simulink library "nmm"  (R2021b)
settings: Solver=VariableStepAuto  StartTime=0.0  StopTime=10.0  RelTol=1e-3
undefined symbols (not defined in the file or in its folder): ENUM_NMMCURRENTSTATE_SLEEP, ENUM_SYSNMMSTA_NORMAL, ENUM_SYSNMMSTA_READYSLEEP, FALSE, KNMM_NoNMIdDebounce_s, KNMM_NrmStaDelay_s, KNMM_RdySlpStaDelay_s, KPMM_HVBattSOCThd_pct, slcm, TRUE, ZERO_INT
libraries: hcu_lib x2, simulink x1
settings Model: Creator=13615  LastModifiedBy=FVT22063
settings SolverCC: AlgebraicLoopSolver=TrustRegion
settings DataIOCC: SaveFormat=Array  SignalLoggingSaveFormat=ModelDataLogs  ReturnWorkspaceOutputs=off
settings OptimizationCC: BlockReduction=off  BooleanDataType=off
settings DebuggingCC: SaveWithParameterizedLinksMsg=none  UnderspecifiedInitializationDetection=Classic  MergeDetectMultiDrivingBlocksExec=none  SignalResolutionControl=TryResolveAllWithWarning  SFMachineParentedDataDiag=warning  ArithmeticOperatorsInVariantConditions=warning
settings HardwareCC: TargetUnknown=on
settings ModelReferenceCC: PropagateSignalLabelsOutOfModel=off
settings SFSimCC: SimUseLocalCustomCode=off  CustomCodeUndefinedFunction=UseInterfaceOnly
settings RTWCC: RTWUseLocalCustomCode=off
settings ConfigComp: CovMetricSettings=dw  CovSaveCumulativeToWorkspaceVar=on  CovSaveSingleToWorkspaceVar=on

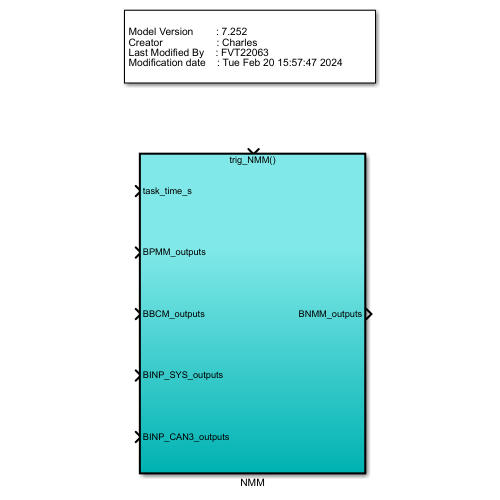
[thumbnail: Simulink's stored preview of the top-level diagram]
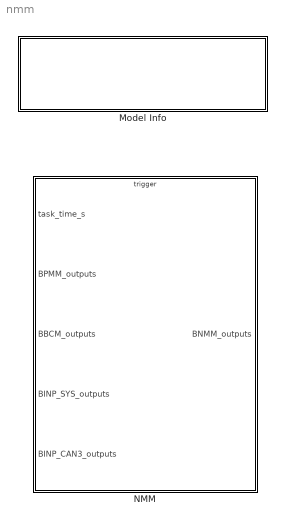
== system nmm ==
  Model Info : Subsystem  LoadFcn=slcm LoadBlock;  InitFcn=slcm('UpdateAllCMBlocksInThisModelInit')  mask(CMBlock){InitialSaveTempField=, InitialBlockCM=None, BlockCM=None, Frame=on, SaveTempField=, DisplayStringWithTags=|, MaskDisplayString=Model Version        : 7.287\nCreator                   : Charles\nLast Modified By    : FVT22063\nModification date    : Tue Aug 27 16:39:44 2024, HorizontalTextAlignment=Left, LeftAlignmentValue=0.02, SourceBlockDiagram=pmm, TagMaxNumber=20, CMTag1=, CMTag2=, CMTag3=, CMTag4=, CMTag5=, CMTag6=, CMTag7=, CMTag8=, CMTag9=, CMTag10=, CMTag11=, CMTag12=, CMTag13=, CMTag14=, CMTag15=, CMTag16=, CMTag17=, CMTag18=, CMTag19=, CMTag20=}
      mask DisplayStringWithTags=|
      | Model Version        : %<ModelVersion>
      | Creator                   : Charles
      | Last Modified By    : %<LastModifiedBy>
      | Modification date    : %<LastModificationDate>
      mask help: This block allows revision control information to be displayed within the model.
      settings: CopyFcn=slcm CopyBlock;  DeleteFcn=slcm Cancel;  PostSaveFcn=slcm('UpdateAllCMBlocksInThisModel')  NameChangeFcn=slcm Rename;  OpenFcn=slcm
      mask Display: text(str2num(LeftAlignmentValue), 0.5, MaskDisplayString, 'HorizontalAlignment', HorizontalTextAlignment)
  NMM : Subsystem  TreatAsAtomicUnit=on
      settings: RTWSystemCode=Nonreusable function  RTWFcnNameOpts=Use subsystem name  RTWFileNameOpts=Use subsystem name

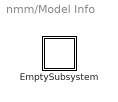
== system nmm/Model Info ==
  EmptySubsystem : Subsystem

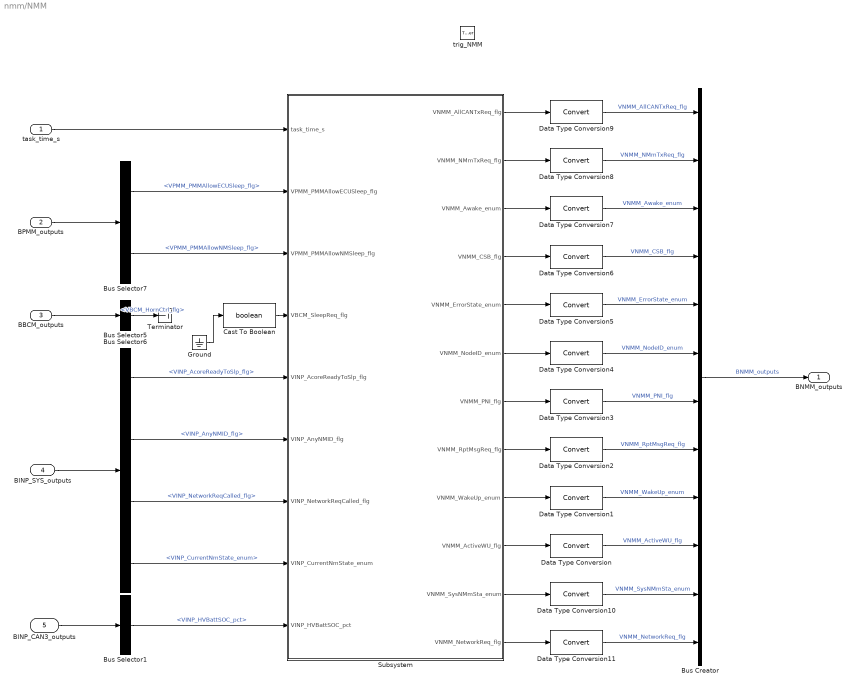
== system nmm/NMM ==
  task_time_s : Inport
  BPMM_outputs : Inport  Port=2  OutDataTypeStr=Bus: BPMM_outputs
  BBCM_outputs : Inport  Port=3  OutDataTypeStr=Bus: BBCM_outputs
  BINP_SYS_outputs : Inport  Port=4  OutDataTypeStr=Bus: BINP_SYS_outputs
  BINP_CAN3_outputs : Inport  Port=5  OutDataTypeStr=Bus: BINP_CAN3_outputs
  trig_NMM : TriggerPort  TriggerType=function-call  VariantControl=(inherit)
  Bus Creator : BusCreator  Inputs=12  OutDataTypeStr=Bus: BNMM_outputs
  Bus Selector1 : BusSelector  OutputSignals=VINP_HVBattSOC_pct
  Bus Selector5 : BusSelector  OutputSignals=VBCM_HornCtrl_flg
  Bus Selector6 : BusSelector  OutputSignals=VINP_AcoreReadyToSlp_flg,VINP_AnyNMID_flg,VINP_NetworkReqCalled_flg,VINP_CurrentNmState_enum
  Bus Selector7 : BusSelector  OutputSignals=VPMM_PMMAllowECUSleep_flg,VPMM_PMMAllowNMSleep_flg
  Cast To Boolean : DataTypeConversion  OutDataTypeStr=boolean
  Data Type Conversion{,1..11} (12 alike) : DataTypeConversion
  Ground : Ground
  Subsystem : Subsystem
  Terminator : Terminator
  BNMM_outputs : Outport  OutDataTypeStr=Bus: BNMM_outputs  LockScale=on
  wires:
  Data Type Conversion9/1 -> Bus Creator/1  "VNMM_AllCANTxReq_flg"
  Data Type Conversion8/1 -> Bus Creator/2  "VNMM_NMmTxReq_flg"
  Data Type Conversion7/1 -> Bus Creator/3  "VNMM_Awake_enum"
  Data Type Conversion6/1 -> Bus Creator/4  "VNMM_CSB_flg"
  Data Type Conversion5/1 -> Bus Creator/5  "VNMM_ErrorState_enum"
  Data Type Conversion4/1 -> Bus Creator/6  "VNMM_NodeID_enum"
  Data Type Conversion3/1 -> Bus Creator/7  "VNMM_PNI_flg"
  Data Type Conversion2/1 -> Bus Creator/8  "VNMM_RptMsgReq_flg"
  Data Type Conversion1/1 -> Bus Creator/9  "VNMM_WakeUp_enum"
  Data Type Conversion/1 -> Bus Creator/10  "VNMM_ActiveWU_flg"
  Bus Creator/1 -> BNMM_outputs/1  "BNMM_outputs"
  Subsystem/10(VNMM_ActiveWU_flg) -> Data Type Conversion/1
  Subsystem/9(VNMM_WakeUp_enum) -> Data Type Conversion1/1
  Subsystem/8(VNMM_RptMsgReq_flg) -> Data Type Conversion2/1
  Subsystem/7(VNMM_PNI_flg) -> Data Type Conversion3/1
  Subsystem/6(VNMM_NodeID_enum) -> Data Type Conversion4/1
  Subsystem/5(VNMM_ErrorState_enum) -> Data Type Conversion5/1
  Subsystem/4(VNMM_CSB_flg) -> Data Type Conversion6/1
  Subsystem/3(VNMM_Awake_enum) -> Data Type Conversion7/1
  Subsystem/2(VNMM_NMmTxReq_flg) -> Data Type Conversion8/1
  Subsystem/1(VNMM_AllCANTxReq_flg) -> Data Type Conversion9/1
  BPMM_outputs/1 -> Bus Selector7/1
  Data Type Conversion10/1 -> Bus Creator/11  "VNMM_SysNMmSta_enum"
  Subsystem/11(VNMM_SysNMmSta_enum) -> Data Type Conversion10/1
  BBCM_outputs/1 -> Bus Selector5/1
  BINP_SYS_outputs/1 -> Bus Selector6/1
  Data Type Conversion11/1 -> Bus Creator/12  "VNMM_NetworkReq_flg"
  Subsystem/12(VNMM_NetworkReq_flg) -> Data Type Conversion11/1
  task_time_s/1 -> Subsystem/1(task_time_s)
  Bus Selector7/2 -> Subsystem/3(VPMM_PMMAllowNMSleep_flg)  "<VPMM_PMMAllowNMSleep_flg>"
  Bus Selector6/2 -> Subsystem/6(VINP_AnyNMID_flg)  "<VINP_AnyNMID_flg>"
  Bus Selector6/1 -> Subsystem/5(VINP_AcoreReadyToSlp_flg)  "<VINP_AcoreReadyToSlp_flg>"
  Bus Selector1/1 -> Subsystem/9(VINP_HVBattSOC_pct)  "<VINP_HVBattSOC_pct>"
  BINP_CAN3_outputs/1 -> Bus Selector1/1
  Bus Selector7/1 -> Subsystem/2(VPMM_PMMAllowECUSleep_flg)  "<VPMM_PMMAllowECUSleep_flg>"
  Bus Selector6/3 -> Subsystem/7(VINP_NetworkReqCalled_flg)  "<VINP_NetworkReqCalled_flg>"
  Bus Selector6/4 -> Subsystem/8(VINP_CurrentNmState_enum)  "<VINP_CurrentNmState_enum>"
  Cast To Boolean/1 -> Subsystem/4(VBCM_SleepReq_flg)
  Ground/1 -> Cast To Boolean/1
  Bus Selector5/1 -> Terminator/1  "<VBCM_HornCtrl_flg>"

== system nmm/Model Info/EmptySubsystem ==

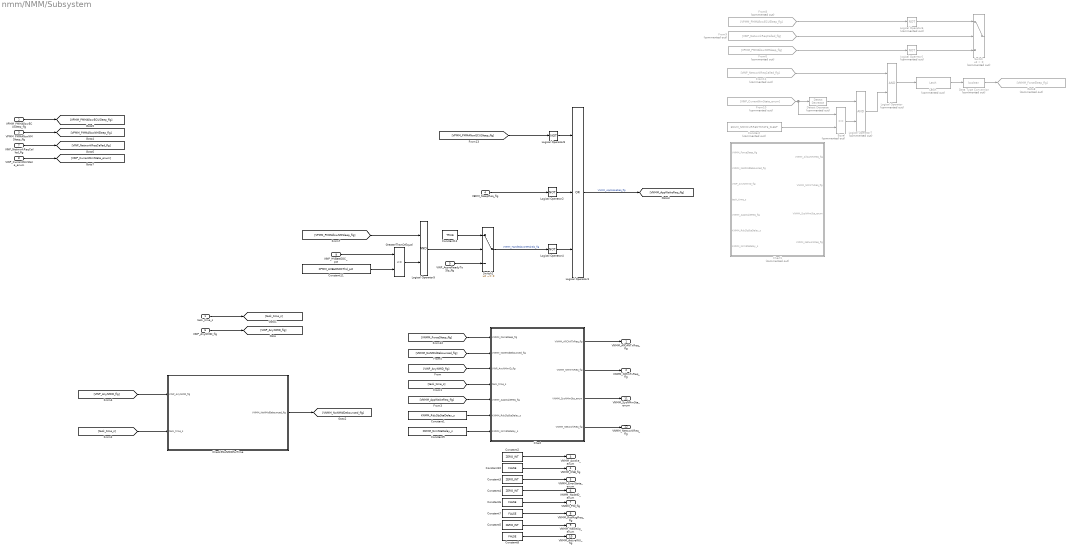
== system nmm/NMM/Subsystem ==
  task_time_s : Inport
  VPMM_PMMAllowECUSleep_flg : Inport  Port=2
  VPMM_PMMAllowNMSleep_flg : Inport  Port=3
  VBCM_SleepReq_flg : Inport  Port=4
  VINP_AcoreReadyToSlp_flg : Inport  Port=5
  VINP_AnyNMID_flg : Inport  Port=6
  VINP_NetworkReqCalled_flg : Inport  Port=7
  VINP_CurrentNmState_enum : Inport  Port=8
  VINP_HVBattSOC_pct : Inport  Port=9
  Chart : Stateflow chart  TreatAsAtomicUnit=on
  Chart1 : Stateflow chart  Commented=on  TreatAsAtomicUnit=on
  CheckIfNoNMIDforTime : Subsystem
  Constant : Constant  Commented=on  Value=ENUM_NMMCURRENTSTATE_SLEEP
  Constant1 : Constant  Value=KNMM_RdySlpStaDelay_s
  Constant{6..8,10} (4 alike) : Constant  Value=FALSE  OutDataTypeStr=boolean
  Constant11 : Constant  Value=KPMM_HVBattSOCThd_pct
  Constant12 : Constant  Value=TRUE
  Constant{2..5} (4 alike) : Constant  Value=ZERO_INT  OutDataTypeStr=uint8
  Constant9 : Constant  Value=KNMM_NrmStaDelay_s
  Data Type Conversion : DataTypeConversion  Commented=on  OutDataTypeStr=boolean
  Detect Decrease : simulink/Logic and Bit Operations/Detect Decrease  Commented=on  vinit=0.0  OutDataTypeStr=boolean
  Equal : RelationalOperator  Commented=on  Operator===  OutDataTypeStr=boolean  RndMeth=Simplest
  From10 : From  Commented=on  GotoTag=VINP_CurrentNmState_enum
  From11 : From  Commented=on  GotoTag=VINP_NetworkReqCalled_flg
  From6 : From  Commented=on  GotoTag=VPMM_PMMAllowNMSleep_flg
  From8 : From  Commented=on  GotoTag=VPMM_PMMAllowECUSleep_flg
  From9 : From  Commented=on  GotoTag=VINP_NetworkReqCalled_flg
  Goto8 : Goto  Commented=on  GotoTag=VNMM_ForceSleep_flg
  GreaterThanOrEqual : RelationalOperator  Operator=<=  OutDataTypeStr=boolean  RndMeth=Simplest
  Latch : hcu_lib/Basic_Blocks/Latch  Commented=on
  Logical Operator : Logic  Commented=on  AllPortsSameDT=off  OutDataTypeStr=boolean
  Logical Operator1 : Logic  Commented=on  Operator=NOT  AllPortsSameDT=off  OutDataTypeStr=boolean
  Logical Operator2 : Logic  Operator=NOT  AllPortsSameDT=off  OutDataTypeStr=boolean
  Logical Operator3 : Logic  Operator=OR  Inputs=3  AllPortsSameDT=off  OutDataTypeStr=boolean
  Logical Operator4 : Logic  Operator=NOT  AllPortsSameDT=off  OutDataTypeStr=boolean
  Logical Operator5 : Logic  AllPortsSameDT=off  OutDataTypeStr=boolean
  Logical Operator6 : Logic  Commented=on  Operator=NOT  AllPortsSameDT=off  OutDataTypeStr=boolean
  Logical Operator7 : Logic  Commented=on  AllPortsSameDT=off  OutDataTypeStr=boolean
  Logical Operator8 : Logic  Operator=NOT  AllPortsSameDT=off  OutDataTypeStr=boolean
  Switch : Switch  Commented=on  Criteria=u2 > Threshold
  Switch2 : Switch  Criteria=u2 ~= 0
  VNMM_AllCANTxReq_flg : Outport
  VNMM_NMmTxReq_flg : Outport  Port=2
  VNMM_Awake_enum : Outport  Port=3
  VNMM_CSB_flg : Outport  Port=4
  VNMM_ErrorState_enum : Outport  Port=5
  VNMM_NodeID_enum : Outport  Port=6
  VNMM_PNI_flg : Outport  Port=7
  VNMM_RptMsgReq_flg : Outport  Port=8
  VNMM_WakeUp_enum : Outport  Port=9
  VNMM_ActiveWU_flg : Outport  Port=10
  VNMM_SysNMmSta_enum : Outport  Port=11
  VNMM_NetworkReq_flg : Outport  Port=12
  wires:
  Constant8/1 -> VNMM_ActiveWU_flg/1
  Constant5/1 -> VNMM_WakeUp_enum/1
  Constant7/1 -> VNMM_RptMsgReq_flg/1
  Constant6/1 -> VNMM_PNI_flg/1
  Constant4/1 -> VNMM_NodeID_enum/1
  Constant3/1 -> VNMM_ErrorState_enum/1
  Constant10/1 -> VNMM_CSB_flg/1
  Constant2/1 -> VNMM_Awake_enum/1
  VBCM_SleepReq_flg/1 -> Logical Operator2/1
  Logical Operator3/1 -> [VNMM_AppWakeReq_flg]  "VNMM_AppWakeReq_flg"
  Logical Operator2/1 -> Logical Operator3/2
  Logical Operator1/1 -> Switch/3
  Logical Operator4/1 -> Logical Operator3/3
  [task_time_s] -> CheckIfNoNMIDforTime/2(task_time_s)
  [VINP_AnyNMID_flg] -> CheckIfNoNMIDforTime/1(VINP_AnyNMID_flg)
  CheckIfNoNMIDforTime/1(VNMM_NoNMIdDebounced_flg) -> [VNMM_NoNMIdDebounced_flg]
  [task_time_s] -> Chart/4(task_time_s)
  task_time_s/1 -> [task_time_s]
  [VINP_AnyNMID_flg] -> Chart/3(VINP_AnyNMmID_flg)
  Constant9/1 -> Chart/7(KNMM_NrmStaDelay_s)
  Constant1/1 -> Chart/6(KNMM_RdySlpStaDelay_s)
  [VNMM_NoNMIdDebounced_flg] -> Chart/2(VNMM_NoNMIdDebounced_flg)
  [VNMM_AppWakeReq_flg] -> Chart/5(VNMM_AppWakeReq_flg)
  VINP_AnyNMID_flg/1 -> [VINP_AnyNMID_flg]
  Chart/3(VNMM_SysNMmSta_enum) -> VNMM_SysNMmSta_enum/1
  Chart/2(VNMM_NMmTxReq_flg) -> VNMM_NMmTxReq_flg/1
  Chart/1(VNMM_AllCANTxReq_flg) -> VNMM_AllCANTxReq_flg/1
  Constant12/1 -> Switch2/1
  VINP_HVBattSOC_pct/1 -> GreaterThanOrEqual/1
  Constant11/1 -> GreaterThanOrEqual/2
  [VPMM_PMMAllowNMSleep_flg] -> Logical Operator5/1
  GreaterThanOrEqual/1 -> Logical Operator5/2
  Logical Operator5/1 -> Switch2/2
  Switch2/1 -> Logical Operator4/1  "VNMM_HandledAcoreRdySlp_flg"
  VINP_AcoreReadyToSlp_flg/1 -> Switch2/3
  From6/1 -> Logical Operator1/1
  VPMM_PMMAllowNMSleep_flg/1 -> [VPMM_PMMAllowNMSleep_flg]
  VPMM_PMMAllowECUSleep_flg/1 -> [VPMM_PMMAllowECUSleep_flg]
  From8/1 -> Logical Operator6/1
  Logical Operator6/1 -> Switch/1
  From9/1 -> Switch/2
  VINP_NetworkReqCalled_flg/1 -> [VINP_NetworkReqCalled_flg]
  VINP_CurrentNmState_enum/1 -> [VINP_CurrentNmState_enum]
  From10/1 -> Detect Decrease/1, Equal/1
  Constant/1 -> Equal/2
  From11/1 -> Logical Operator/1
  Logical Operator7/1 -> Logical Operator/2
  Chart/4(VNMM_NetworkReq_flg) -> VNMM_NetworkReq_flg/1
  [VNMM_ForceSleep_flg] -> Chart/1(VNMM_ForceSleep_flg)
  Logical Operator/1 -> Latch/1
  Detect Decrease/1 -> Logical Operator7/1
  Equal/1 -> Logical Operator7/2
  Latch/1 -> Data Type Conversion/1
  Data Type Conversion/1 -> Goto8/1
  [VPMM_PMMAllowECUSleep_flg] -> Logical Operator8/1
  Logical Operator8/1 -> Logical Operator3/1

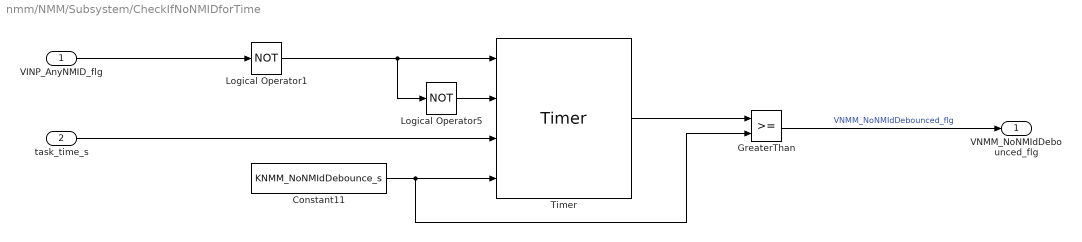
== system nmm/NMM/Subsystem/CheckIfNoNMIDforTime ==
  VINP_AnyNMID_flg : Inport
  task_time_s : Inport  Port=2
  Constant11 : Constant  Value=KNMM_NoNMIdDebounce_s
  GreaterThan : RelationalOperator  OutDataTypeStr=boolean  RndMeth=Simplest
  Logical Operator1 : Logic  Operator=NOT  AllPortsSameDT=off  OutDataTypeStr=boolean
  Logical Operator5 : Logic  Operator=NOT  AllPortsSameDT=off  OutDataTypeStr=boolean
  Timer : hcu_lib/Basic_Blocks/Timer
  VNMM_NoNMIdDebounced_flg : Outport
  wires:
  Logical Operator5/1 -> Timer/2
  VINP_AnyNMID_flg/1 -> Logical Operator1/1
  Constant11/1 -> GreaterThan/2, Timer/4
  task_time_s/1 -> Timer/3
  Timer/1 -> GreaterThan/1
  GreaterThan/1 -> VNMM_NoNMIdDebounced_flg/1  "VNMM_NoNMIdDebounced_flg"
  Logical Operator1/1 -> Logical Operator5/1, Timer/1

== stateflow chart nmm/NMM/Subsystem/Chart1 ==
  state State_Machine
    en:
    VNMM_AllCANTxReq_flg = TRUE;
    VNMM_NMmTxReq_flg = TRUE;
    state Normal_State
      en:
      VNMM_SysNMmSta_enum = ENUM_SYSNMMSTA_NORMAL;
      VNMM_NetworkReq_flg = TRUE;
      %VNMM_NrmStaDelayDone_flg =FALSE;
      (default) -> (junction 90) [commented out] : {VNMM_NrmStaDelayTimer_s = 0;}
      Normal_State -> (junction 90) [commented out]
      (junction 90) -> (junction 97) [commented out] : [VNMM_NrmStaDelayTimer_s >= KNMM_NrmStaDelay_s]
      (junction 90) -> (junction 95) [commented out] : {VNMM_NrmStaDelayTimer_s += task_time_s;}
      (junction 97) -> (junction 99) [commented out] : {VNMM_NrmStaDelayDone_flg = TRUE;}
      (junction 99) -> (junction 95) [commented out]
    state Ready_Sleep
      en:
      VNMM_SysNMmSta_enum = ENUM_SYSNMMSTA_READYSLEEP;
      VNMM_NetworkReq_flg = FALSE;
      //VNMM_RdySlpStaDelayDone_flg = FALSE;
      (default) -> (junction 108) [commented out] : {VNMM_RdySlpStaDelayTimer_s = 0;}
      Ready_Sleep -> (junction 108) [commented out]
      (junction 108) -> (junction 111) [commented out] : [VNMM_RdySlpStaDelayTimer_s >= KNMM_RdySlpStaDelay_s]
      (junction 108) -> (junction 114) [commented out] : {VNMM_RdySlpStaDelayTimer_s += task_time_s;}
      (junction 111) -> (junction 110) [commented out] : {VNMM_RdySlpStaDelayDone_flg = TRUE;}
      (junction 110) -> (junction 114) [commented out]
    (default) -> (junction 123)
    (junction 123) -> Normal_State [order 1] : [
        |  //VNMM_RdySlpStaDelayDone_flg &&...
        |  (VINP_AnyNMmID_flg ||...
        |   VNMM_AppWakeReq_flg) &&...
        |  !VNMM_ForceSleep_flg
        | ]
    (junction 123) -> (junction 121) [order 2]
    Ready_Sleep -> Normal_State : [
        |  //VNMM_RdySlpStaDelayDone_flg &&...
        |  (VINP_AnyNMmID_flg ||...
        |   VNMM_AppWakeReq_flg) &&...
        |  !VNMM_ForceSleep_flg
        | ]
    Normal_State -> Ready_Sleep : [
        |  (VNMM_NoNMIdDebounced_flg && ...
        |   !VNMM_AppWakeReq_flg) ||...
        |  VNMM_ForceSleep_flg
        | ]
    (junction 121) -> Ready_Sleep
  (default) -> State_Machine
  data: VNMM_ForceSleep_flg input; VNMM_NoNMIdDebounced_flg input; VNMM_AllCANTxReq_flg output boolean; VINP_AnyNMmID_flg input; task_time_s input; TRUE parameter; FALSE parameter; VNMM_NMmTxReq_flg output boolean; VNMM_AppWakeReq_flg input; ENUM_SYSNMMSTA_READYSLEEP parameter; ENUM_SYSNMMSTA_NORMAL parameter; VNMM_SysNMmSta_enum output uint8; VNMM_NetworkReq_flg output boolean; VNMM_NrmStaDelayDone_flg local boolean; VNMM_NrmStaDelayTimer_s local single; VNMM_RdySlpStaDelayDone_flg local boolean; VNMM_RdySlpStaDelayTimer_s local single; KNMM_RdySlpStaDelay_s input; KNMM_NrmStaDelay_s input

== stateflow chart nmm/NMM/Subsystem/Chart ==
  state State_Machine
    en:
    VNMM_AllCANTxReq_flg = TRUE;
    VNMM_NMmTxReq_flg = TRUE;
    state Normal_State
      en:
      VNMM_SysNMmSta_enum = ENUM_SYSNMMSTA_NORMAL;
      VNMM_NetworkReq_flg = TRUE;
      %VNMM_NrmStaDelayDone_flg =FALSE;
      (default) -> (junction 90) [commented out] : {VNMM_NrmStaDelayTimer_s = 0;}
      Normal_State -> (junction 90) [commented out]
      (junction 90) -> (junction 97) [commented out] : [VNMM_NrmStaDelayTimer_s >= KNMM_NrmStaDelay_s]
      (junction 90) -> (junction 95) [commented out] : {VNMM_NrmStaDelayTimer_s += task_time_s;}
      (junction 97) -> (junction 99) [commented out] : {VNMM_NrmStaDelayDone_flg = TRUE;}
      (junction 99) -> (junction 95) [commented out]
    state Ready_Sleep
      en:
      VNMM_SysNMmSta_enum = ENUM_SYSNMMSTA_READYSLEEP;
      VNMM_NetworkReq_flg = FALSE;
      //VNMM_RdySlpStaDelayDone_flg = FALSE;
      (default) -> (junction 108) [commented out] : {VNMM_RdySlpStaDelayTimer_s = 0;}
      Ready_Sleep -> (junction 108) [commented out]
      (junction 108) -> (junction 111) [commented out] : [VNMM_RdySlpStaDelayTimer_s >= KNMM_RdySlpStaDelay_s]
      (junction 108) -> (junction 114) [commented out] : {VNMM_RdySlpStaDelayTimer_s += task_time_s;}
      (junction 111) -> (junction 110) [commented out] : {VNMM_RdySlpStaDelayDone_flg = TRUE;}
      (junction 110) -> (junction 114) [commented out]
    (default) -> Normal_State
    Ready_Sleep -> Normal_State : [
        |  //VNMM_RdySlpStaDelayDone_flg &&...
        |   VINP_AnyNMmID_flg ||...
        |   VNMM_AppWakeReq_flg
        | ]
    Normal_State -> Ready_Sleep : [
        |   VNMM_NoNMIdDebounced_flg && ...
        |   !VNMM_AppWakeReq_flg
        | ]
  (default) -> State_Machine
  data: VNMM_ForceSleep_flg input; VNMM_NoNMIdDebounced_flg input; VNMM_AllCANTxReq_flg output boolean; VINP_AnyNMmID_flg input; task_time_s input; TRUE parameter; FALSE parameter; VNMM_NMmTxReq_flg output boolean; VNMM_AppWakeReq_flg input; ENUM_SYSNMMSTA_READYSLEEP parameter; ENUM_SYSNMMSTA_NORMAL parameter; VNMM_SysNMmSta_enum output uint8; VNMM_NetworkReq_flg output boolean; VNMM_NrmStaDelayDone_flg local boolean; VNMM_NrmStaDelayTimer_s local single; VNMM_RdySlpStaDelayDone_flg local boolean; VNMM_RdySlpStaDelayTimer_s local single; KNMM_RdySlpStaDelay_s input; KNMM_NrmStaDelay_s input
